simulink model "TP_8"  (R2023b)
settings: Solver=VariableStepAuto  StartTime=0.0  StopTime=10.0  RelTol=1e-3
libraries: spsThyristorLib x2, spsACVoltageSourceLib x1, spsSeriesRLCBranchLib x1, spsVariableRatioTransformerLib x1
settings Model: Creator=sohayl  LastModifiedBy=sohayl

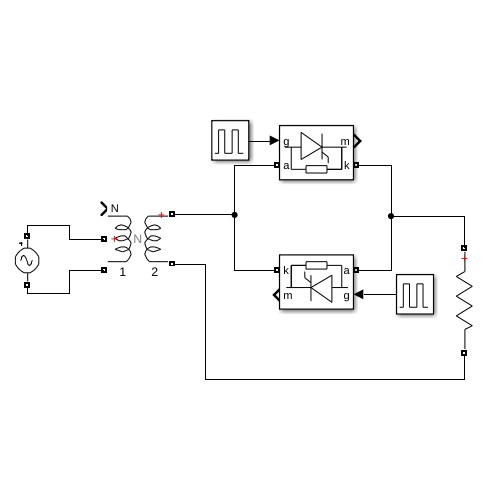
[thumbnail: Simulink's stored preview of the top-level diagram]
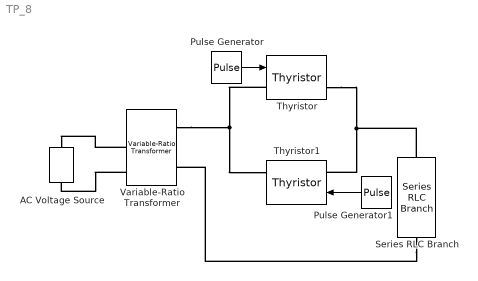
== system TP_8 ==
  AC Voltage Source : spsACVoltageSourceLib/AC Voltage Source  Amplitude=24  Phase=0  Frequency=50  SampleTime=0  Measurements=None  BusType=swing  Pref=10e3  Qref=0  Qmin=-inf  Qmax=+inf
  Pulse Generator : DiscretePulseGenerator  PulseType=Time based  Period=10  PulseWidth=5
  Pulse Generator1 : DiscretePulseGenerator  PulseType=Time based  Period=10  PulseWidth=5
  Series RLC Branch : spsSeriesRLCBranchLib/Series RLC Branch  LConnTagsString=__new0  RConnTagsString=__new0  BranchType=R  Resistance=500  Inductance=1e-3  SetiL0=off  InitialCurrent=0  Capacitance=1e-6  Setx0=off  InitialVoltage=0  Measurements=None
  Thyristor : spsThyristorLib/Thyristor  Ron=0.001  Lon=0  Vf=0.8  IC=0  Rs=500  Cs=250e-9  Measurements=on
  Thyristor1 : spsThyristorLib/Thyristor  Ron=0.001  Lon=0  Vf=0.8  IC=0  Rs=500  Cs=250e-9  Measurements=on
  Variable-Ratio Transformer : spsVariableRatioTransformerLib/Variable-Ratio Transformer
      settings: LibrarySourceBlock=|
      | sps_lib/Passives/Variable-Ratio
      | Transformer
  wires:
  Pulse Generator/1 -> Thyristor/1
  Pulse Generator1/1 -> Thyristor1/1
  connections:
  Variable-Ratio Transformer/LConn1 -- AC Voltage Source/RConn1
  Variable-Ratio Transformer/LConn2 -- AC Voltage Source/LConn1
  Thyristor/RConn1 -- Series RLC Branch/LConn1 -- Thyristor1/LConn1
  Thyristor/LConn1 -- Variable-Ratio Transformer/RConn1 -- Thyristor1/RConn1
  Series RLC Branch/RConn1 -- Variable-Ratio Transformer/RConn2
